simulink model "Laplace_Time_Shift"  (R2024b)
settings: Solver=VariableStepAuto  StartTime=0.0  StopTime=10.0  RelTol=1e-3
settings Model: Creator=user  LastModifiedBy=user

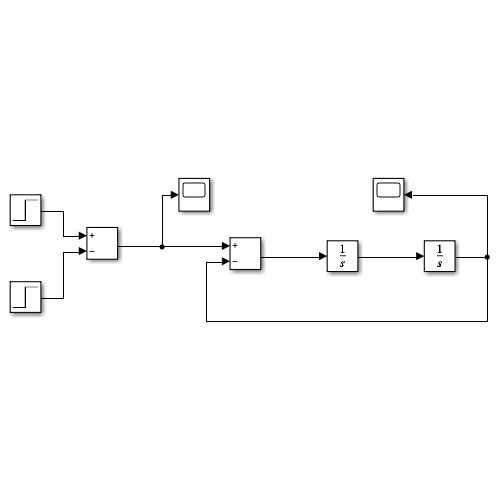
[thumbnail: Simulink's stored preview of the top-level diagram]
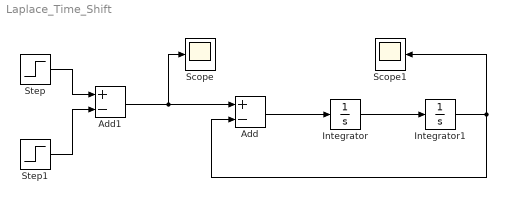
== system Laplace_Time_Shift ==
  Add : Sum  Inputs=+-
  Add1 : Sum  Inputs=+-
  Integrator : Integrator
  Integrator1 : Integrator
  Scope : Scope
  Scope1 : Scope
  Step : Step  SampleTime=0
  Step1 : Step  Time=5  SampleTime=0
  wires:
  Integrator/1 -> Integrator1/1
  Add/1 -> Integrator/1
  Step/1 -> Add1/1
  Step1/1 -> Add1/2
  Add1/1 -> Scope/1, Add/1
  Integrator1/1 -> Scope1/1, Add/2
